simulink model "PMSM_Simulation"  (R2023a)
settings: Solver=ode23t  StartTime=0.0  StopTime=5  MaxStep=0.2  RelTol=1e-4  EnableMultiTasking=on
InitFcn:
  | p = 4;
  | Ld = 0.000425;
  | Lq = 0.00085;
  | psim = 0.119489;
  | Rs = 0.0485;
  | J = 0.00027;
  | Kpwm = 1;
  | Tsi = 0.0001;
  | h = 900;
  | 
  | L0 = (Ld+Lq)/2;
  | SMO_Kp = 100;
  | SMO_Coef =0.0001;
  | Ki_id = Ld*(h+1)/(4.5*Kpwm*(Tsi^2)*(h^2));
  | Kp_id = Ld*(h+1)/(4.5*Kpwm*Tsi*h);
  | 
  | wc =3000;
  | 
  | Ki_iq = Lq*(h+1)/(4.5*Kpwm*Tsi^2*h^2);
  | Kp_iq = Lq*(h+1)/(4.5*Kpwm*Tsi*h);
  | 
  | 
  | Kp_Spd = pi*J/(300*p*psim*Tsi)
  | Ki_Spd = pi*J/(6000*p*psim*Tsi^2)
  | 
  | DeadTime = 2e-6;
  | 
  | Udc = 650;
model workspace (MAT data in the model file):
  KfDeadCompen_CpPeriodTimesT_NULL : Simulink.Parameter (value not decoded)
  KfMDCC_InvParkCpPeriodTimesT_NULL : Simulink.Parameter (value not decoded)
values from neighbouring files (symbols this model uses):
  KfDeadCompen_SetDeltaTime_us = myPackage.Parameter    [DeadCompen.m]
  VbDeadComp_SwtUseIsttrDes_flg = myPackage.Parameter    [DeadCompen.m]
  VfDeadCompen_agIPredAdpr_C = myPackage.Parameter    [DeadCompen.m]
  VfDeadCompen_ISttrDdeThdSwt_A = myPackage.Parameter    [DeadCompen.m]
  VfDeadCompen_ISttrIgbtThdSwt_A = myPackage.Parameter    [DeadCompen.m]
  VfDeadCompen_rDdeISttrHi_R = myPackage.Parameter    [DeadCompen.m]
  VfDeadCompen_rDdeISttrLo_R = myPackage.Parameter    [DeadCompen.m]
  VfDeadCompen_rIgbtISttrHi_R = myPackage.Parameter    [DeadCompen.m]
  VfDeadCompen_rIgbtISttrLo_R = myPackage.Parameter    [DeadCompen.m]
  VfDeadCompen_uDdeISttrHi_V = myPackage.Parameter    [DeadCompen.m]
  VfDeadCompen_uDdeISttrLo_V = myPackage.Parameter    [DeadCompen.m]
  VfDeadCompen_uIgbtISttrHi_V = myPackage.Parameter    [DeadCompen.m]
  VfDeadCompen_uIgbtISttrLo_V = myPackage.Parameter    [DeadCompen.m]
symbols that are objects in the model workspace (value not decoded): KfDeadCompen_CpPeriodTimesT_NULL, KfMDCC_InvParkCpPeriodTimesT_NULL
undefined symbols (not defined in the file or in its folder): DiscIntNeverNeededParam, TableDeadTime_us, TableDeadTimeLookUpCur_A, VuDeadCompen_agIPredAdpr_C
libraries: simulink x23, mcbcontrolslib x11, mcbplantlib x1, spsCurrentMeasurementLib x1, spsDCVoltageSourceLib x1, spsMultimeterLib x1, spsPermanentMagnetSynchronousMachineLib x1, eePmsmCurrentController x1, spsThreePhaseVIMeasurementLib x1, spsUniversalBridgeLib x1, spspowerguiLib x1
(part 4 of 4)

== system PMSM_Simulation/Subsystem/Subsystem/DeadComp_Sys/Subsystem/Tavon_Calc/ia2/uIgbtCalc/If Action Subsystem1 ==
  iPhaseAbs : Inport
  Action Port : ActionPort
  Add : Sum
  Constant : Constant  Value=VfDeadCompen_uIgbtISttrHi_V
  Constant1 : Constant  Value=VfDeadCompen_rIgbtISttrHi_R
  Product : Product
  uIgbt : Outport
  wires:
  iPhaseAbs/1 -> Product/2
  Constant/1 -> Add/1
  Add/1 -> uIgbt/1
  Constant1/1 -> Product/1
  Product/1 -> Add/2

== system PMSM_Simulation/Subsystem/Subsystem/Subsystem2/Subsystem/Tavon_Calc/ia/uDdeCalc/If Action Subsystem ==
  iPhaseAbs : Inport
  Action Port : ActionPort  ActionPortLabel=if(u1 == 1)
  Add : Sum
  Constant : Constant  Value=VfDeadCompen_uDdeISttrLo_V
  Constant1 : Constant  Value=VfDeadCompen_rDdeISttrLo_R
  Product : Product
  UDde : Outport
  wires:
  Constant/1 -> Add/1
  Constant1/1 -> Product/1
  iPhaseAbs/1 -> Product/2
  Product/1 -> Add/2
  Add/1 -> UDde/1

== system PMSM_Simulation/Subsystem/Subsystem/Subsystem2/Subsystem/Tavon_Calc/ia/uDdeCalc/If Action Subsystem1 ==
  iPhaseAbs : Inport
  Action Port : ActionPort  ActionPortLabel=else
  Add : Sum
  Constant : Constant  Value=VfDeadCompen_uDdeISttrHi_V
  Constant1 : Constant  Value=VfDeadCompen_rDdeISttrHi_R
  Product : Product
  UDde : Outport
  wires:
  iPhaseAbs/1 -> Product/2
  Constant/1 -> Add/1
  Add/1 -> UDde/1
  Constant1/1 -> Product/1
  Product/1 -> Add/2

== system PMSM_Simulation/Subsystem/Subsystem/Subsystem2/Subsystem/Tavon_Calc/ia/uIgbtCalc/If Action Subsystem ==
  iPhaseAbs : Inport
  Action Port : ActionPort  ActionPortLabel=if(u1 == 0)
  Add : Sum
  Constant : Constant  Value=VfDeadCompen_uIgbtISttrLo_V
  Constant1 : Constant  Value=VfDeadCompen_rIgbtISttrLo_R
  Product : Product
  uIgbt : Outport
  wires:
  Constant/1 -> Add/1
  Constant1/1 -> Product/1
  iPhaseAbs/1 -> Product/2
  Product/1 -> Add/2
  Add/1 -> uIgbt/1

== system PMSM_Simulation/Subsystem/Subsystem/Subsystem2/Subsystem/Tavon_Calc/ia/uIgbtCalc/If Action Subsystem1 ==
  iPhaseAbs : Inport
  Action Port : ActionPort  ActionPortLabel=else
  Add : Sum
  Constant : Constant  Value=VfDeadCompen_uIgbtISttrHi_V
  Constant1 : Constant  Value=VfDeadCompen_rIgbtISttrHi_R
  Product : Product
  uIgbt : Outport
  wires:
  iPhaseAbs/1 -> Product/2
  Constant/1 -> Add/1
  Add/1 -> uIgbt/1
  Constant1/1 -> Product/1
  Product/1 -> Add/2

== system PMSM_Simulation/Subsystem/Subsystem/Subsystem2/Subsystem/Tavon_Calc/ia1/uDdeCalc/If Action Subsystem ==
  iPhaseAbs : Inport
  Action Port : ActionPort  ActionPortLabel=if(u1 == 1)
  Add : Sum
  Constant : Constant  Value=VfDeadCompen_uDdeISttrLo_V
  Constant1 : Constant  Value=VfDeadCompen_rDdeISttrLo_R
  Product : Product
  UDde : Outport
  wires:
  Constant/1 -> Add/1
  Constant1/1 -> Product/1
  iPhaseAbs/1 -> Product/2
  Product/1 -> Add/2
  Add/1 -> UDde/1

== system PMSM_Simulation/Subsystem/Subsystem/Subsystem2/Subsystem/Tavon_Calc/ia1/uDdeCalc/If Action Subsystem1 ==
  iPhaseAbs : Inport
  Action Port : ActionPort  ActionPortLabel=else
  Add : Sum
  Constant : Constant  Value=VfDeadCompen_uDdeISttrHi_V
  Constant1 : Constant  Value=VfDeadCompen_rDdeISttrHi_R
  Product : Product
  UDde : Outport
  wires:
  iPhaseAbs/1 -> Product/2
  Constant/1 -> Add/1
  Add/1 -> UDde/1
  Constant1/1 -> Product/1
  Product/1 -> Add/2

== system PMSM_Simulation/Subsystem/Subsystem/Subsystem2/Subsystem/Tavon_Calc/ia1/uIgbtCalc/If Action Subsystem ==
  iPhaseAbs : Inport
  Action Port : ActionPort  ActionPortLabel=if(u1 == 0)
  Add : Sum
  Constant : Constant  Value=VfDeadCompen_uIgbtISttrLo_V
  Constant1 : Constant  Value=VfDeadCompen_rIgbtISttrLo_R
  Product : Product
  uIgbt : Outport
  wires:
  Constant/1 -> Add/1
  Constant1/1 -> Product/1
  iPhaseAbs/1 -> Product/2
  Product/1 -> Add/2
  Add/1 -> uIgbt/1

== system PMSM_Simulation/Subsystem/Subsystem/Subsystem2/Subsystem/Tavon_Calc/ia1/uIgbtCalc/If Action Subsystem1 ==
  iPhaseAbs : Inport
  Action Port : ActionPort  ActionPortLabel=else
  Add : Sum
  Constant : Constant  Value=VfDeadCompen_uIgbtISttrHi_V
  Constant1 : Constant  Value=VfDeadCompen_rIgbtISttrHi_R
  Product : Product
  uIgbt : Outport
  wires:
  iPhaseAbs/1 -> Product/2
  Constant/1 -> Add/1
  Add/1 -> uIgbt/1
  Constant1/1 -> Product/1
  Product/1 -> Add/2

== system PMSM_Simulation/Subsystem/Subsystem/Subsystem2/Subsystem/Tavon_Calc/ia2/uDdeCalc/If Action Subsystem ==
  iPhaseAbs : Inport
  Action Port : ActionPort  ActionPortLabel=if(u1 == 1)
  Add : Sum
  Constant : Constant  Value=VfDeadCompen_uDdeISttrLo_V
  Constant1 : Constant  Value=VfDeadCompen_rDdeISttrLo_R
  Product : Product
  UDde : Outport
  wires:
  Constant/1 -> Add/1
  Constant1/1 -> Product/1
  iPhaseAbs/1 -> Product/2
  Product/1 -> Add/2
  Add/1 -> UDde/1

== system PMSM_Simulation/Subsystem/Subsystem/Subsystem2/Subsystem/Tavon_Calc/ia2/uDdeCalc/If Action Subsystem1 ==
  iPhaseAbs : Inport
  Action Port : ActionPort  ActionPortLabel=else
  Add : Sum
  Constant : Constant  Value=VfDeadCompen_uDdeISttrHi_V
  Constant1 : Constant  Value=VfDeadCompen_rDdeISttrHi_R
  Product : Product
  UDde : Outport
  wires:
  iPhaseAbs/1 -> Product/2
  Constant/1 -> Add/1
  Add/1 -> UDde/1
  Constant1/1 -> Product/1
  Product/1 -> Add/2

== system PMSM_Simulation/Subsystem/Subsystem/Subsystem2/Subsystem/Tavon_Calc/ia2/uIgbtCalc/If Action Subsystem ==
  iPhaseAbs : Inport
  Action Port : ActionPort  ActionPortLabel=if(u1 == 0)
  Add : Sum
  Constant : Constant  Value=VfDeadCompen_uIgbtISttrLo_V
  Constant1 : Constant  Value=VfDeadCompen_rIgbtISttrLo_R
  Product : Product
  uIgbt : Outport
  wires:
  Constant/1 -> Add/1
  Constant1/1 -> Product/1
  iPhaseAbs/1 -> Product/2
  Product/1 -> Add/2
  Add/1 -> uIgbt/1

== system PMSM_Simulation/Subsystem/Subsystem/Subsystem2/Subsystem/Tavon_Calc/ia2/uIgbtCalc/If Action Subsystem1 ==
  iPhaseAbs : Inport
  Action Port : ActionPort  ActionPortLabel=else
  Add : Sum
  Constant : Constant  Value=VfDeadCompen_uIgbtISttrHi_V
  Constant1 : Constant  Value=VfDeadCompen_rIgbtISttrHi_R
  Product : Product
  uIgbt : Outport
  wires:
  iPhaseAbs/1 -> Product/2
  Constant/1 -> Add/1
  Add/1 -> uIgbt/1
  Constant1/1 -> Product/1
  Product/1 -> Add/2

== stateflow chart PMSM_Simulation/Subsystem/Task Scheduler ==
  (default) -> (junction 23) : CLK_50us
  (junction 23) -> (junction 17)
  (junction 17) -> (junction 22) [order 2]
  (junction 17) -> (junction 22) [order 1] : [cnt%%2==0]{Task_100us_1;}
  (junction 22) -> (junction 18) [order 2]
  (junction 22) -> (junction 18) [order 1] : [cnt%%2==0]{Task_100us_2;}
  (junction 18) -> (junction 21) [order 1] : [cnt%%20==0]{Task_1ms_1;}
  (junction 18) -> (junction 21) [order 2]
  (junction 21) -> (junction 34) [order 2]
  (junction 21) -> (junction 16) [order 1] : [1]{cnt++;}
  data: cnt local int32
  events: Task_100us_1 output FUNCTION_CALL_EVENT; Task_100us_2 output FUNCTION_CALL_EVENT; Task_1ms_1 output FUNCTION_CALL_EVENT; CLK_50us input FUNCTION_CALL_EVENT
